simulink model "a3__AM_on_AWGN_channel"  (R2019a)
settings: Solver=VariableStepAuto  StartTime=0.0  StopTime=10.0  RelTol=1e-3
undefined symbols (not defined in the file): magnitude
libraries: dspstat3 x2, commchan3 x1, dsparch4 x1
settings Model: Creator=Thanh_Hai  LastModifiedBy=Thanh_Hai

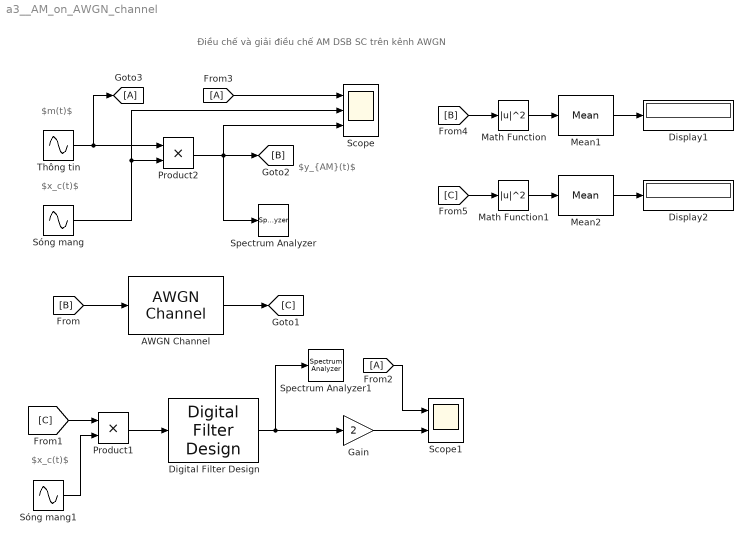
== system a3__AM_on_AWGN_channel ==
  note: $y_{AM}(t)$
  note: $x_c(t)$
  note: $x_c(t)$
  note: $m(t)$
  note: Điều chế và giải điều chế AM DSB SC trên kênh AWGN
  AWGN Channel : commchan3/AWGN Channel  InputProcessing=Columns as channels (frame based)  seed=67  noiseMode=Variance from mask  EbNodB=10  EsNodB=10  SNRdB=10  bitsPerSym=1  Ps=1  Tsym=1  variance=1
      settings: SourceProductName=Communications Toolbox
  Digital Filter Design : dsparch4/Digital Filter Design  mwdsp_browser_bugfix_var=off
  Display1 : Display
  Display2 : Display
  Gain : Gain  Gain=2
  Math Function : Math  Operator=magnitude^2  SaturateOnIntegerOverflow=on
  Math Function1 : Math  Operator=magnitude^2  SaturateOnIntegerOverflow=on
  Mean1 : dspstat3/Mean  run=on  InputProcessing=Columns as channels (frame based)  reset_popup=None  directionMode=Entire input  dimension=1  roiEnable=off  roiType=Rectangles  roiPortion=Entire ROI  roiOutput=Individual statistics for each ROI  roiFlag=off  roundingMode=Floor  overflowMode=off  outputDataTypeStr=Inherit: Same as accumulator  outputMin=[]  outputMax=[]  outputLastDataTypeStr=Inherit: Same as accumulator
  Mean2 : dspstat3/Mean  run=on  InputProcessing=Columns as channels (frame based)  reset_popup=None  directionMode=Entire input  dimension=1  roiEnable=off  roiType=Rectangles  roiPortion=Entire ROI  roiOutput=Individual statistics for each ROI  roiFlag=off  roundingMode=Floor  overflowMode=off  outputDataTypeStr=Inherit: Same as accumulator  outputMin=[]  outputMax=[]  outputLastDataTypeStr=Inherit: Same as accumulator
  Product1 : Product
  Product2 : Product
  Scope : Scope  NumInputPorts=3
  Scope1 : Scope  NumInputPorts=2
  Spectrum Analyzer : SpectrumAnalyzer
  Spectrum Analyzer1 : SpectrumAnalyzer
  Sóng mang : Sin  Frequency=2*pi*5000  SampleTime=1/50000
  Sóng mang1 : Sin  Frequency=2*pi*5000  SampleTime=1/50000
  Thông tin : Sin  Frequency=2*pi*200  SampleTime=1/50000
  wires:
  Product1/1 -> Digital Filter Design/1
  Product2/1 -> Spectrum Analyzer/1, Scope/3, [B]
  [A] -> Scope/1
  Digital Filter Design/1 -> Gain/1, Spectrum Analyzer1/1
  Sóng mang1/1 -> Product1/2
  [A] -> Scope1/1
  Sóng mang/1 -> Scope/2, Product2/2
  Thông tin/1 -> Product2/1, [A]
  Gain/1 -> Scope1/2
  [B] -> AWGN Channel/1
  AWGN Channel/1 -> [C]
  [C] -> Product1/1
  Math Function/1 -> Mean1/1
  [B] -> Math Function/1
  Mean1/1 -> Display1/1
  [C] -> Math Function1/1
  Mean2/1 -> Display2/1
  Math Function1/1 -> Mean2/1
